simulink model "BLOC_Clutch"  (R2016a)
settings: Solver=FixedStepDiscrete  StartTime=0.0  StopTime=10.0  FixedStep=hev_dt  RelTol=1e-3
undefined symbols (not defined in the file): DiscIntNeverNeededParam, fa_clu_pos, fa_clu_pv, fa_ice_inertia, fa_max_tq_clu, hev_dt
libraries: simulink x1
settings Model: Creator=Florent  LastModifiedBy=Florent
settings OptimizationCC: DefaultParameterBehavior=Inlined  OptimizeModelRefInitCode=on  LifeSpan=1
settings RTWCC: SystemTargetFile=ert.tlc  TemplateMakefile=ert_default_tmf  GenerateReport=on  IncludeHyperlinkInReport=on  LaunchReport=on  TargetLang=C++  GenerateTraceInfo=on  GenerateTraceReport=on  GenerateTraceReportSl=on  GenerateTraceReportSf=on  GenerateTraceReportEml=on
settings CodeAppCC: ForceParamTrailComments=on  OperatorAnnotations=on  SimulinkDataObjDesc=on  SFDataObjDesc=on  MATLABFcnDesc=on  InsertBlockDesc=on  MATLABSourceComments=on
settings ERTTargetCC: GenerateSampleERTMain=on  MultiInstanceERTCode=on  CodeInterfacePackaging=C++ class  InlinedParameterPlacement=NonHierarchical  RootIOFormat=Structure reference  ERTCustomFileTemplate=example_file_process.tlc

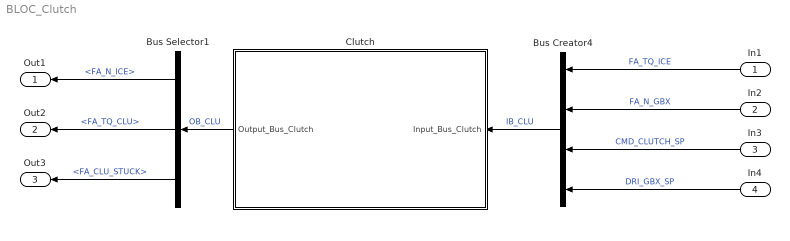
== system BLOC_Clutch ==
  In1 : Inport
  In2 : Inport  Port=2
  In3 : Inport  Port=3
  In4 : Inport  Port=4
  Bus Creator4 : BusCreator  Inputs=4
  Bus Selector1 : BusSelector  OutputSignals=FA_N_ICE,FA_TQ_CLU,FA_CLU_STUCK
  Clutch : Subsystem  TreatAsAtomicUnit=on  SystemSampleTime=hev_dt
  Out1 : Outport
  Out2 : Outport  Port=2
  Out3 : Outport  Port=3
  wires:
  In2/1 -> Bus Creator4/2  "FA_N_GBX"
  In1/1 -> Bus Creator4/1  "FA_TQ_ICE"
  In3/1 -> Bus Creator4/3  "CMD_CLUTCH_SP"
  In4/1 -> Bus Creator4/4  "DRI_GBX_SP"
  Bus Creator4/1 -> Clutch/1("Input_Bus_Clutch ")  "IB_CLU"
  Bus Selector1/2 -> Out2/1  "<FA_TQ_CLU>"
  Clutch/1(Output_Bus_Clutch) -> Bus Selector1/1  "OB_CLU"
  Bus Selector1/3 -> Out3/1  "<FA_CLU_STUCK>"
  Bus Selector1/1 -> Out1/1  "<FA_N_ICE>"

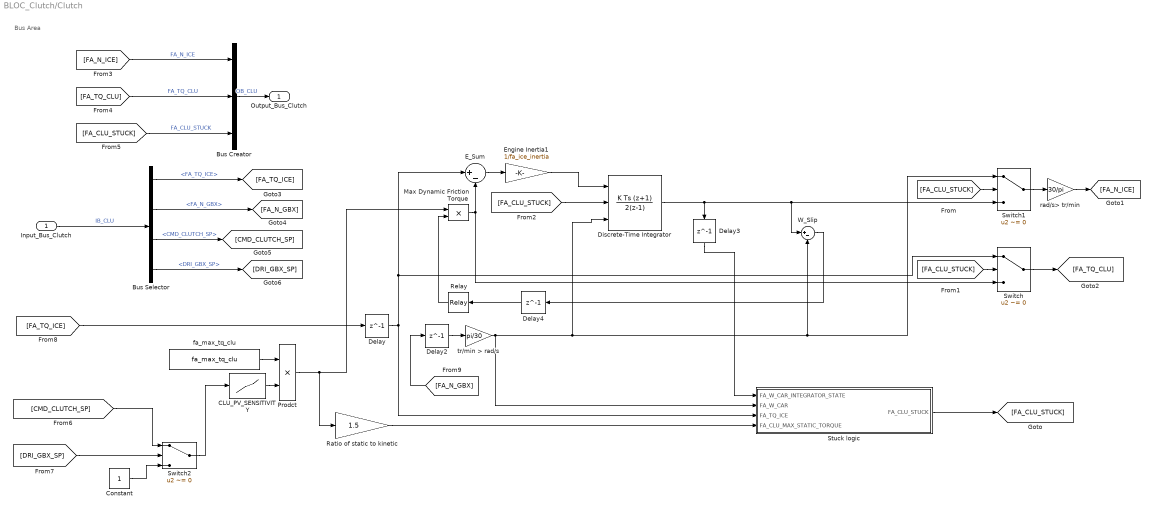
== system BLOC_Clutch/Clutch ==
  note: Bus Area
  "Input_Bus_Clutch " : Inport
  " tr/min > rad/s" : Gain  Gain=pi/30  SampleTime=hev_dt
  Bus Creator : BusCreator  Inputs=3
  Bus Selector : BusSelector  OutputSignals=FA_TQ_ICE,FA_N_GBX,CMD_CLUTCH_SP,DRI_GBX_SP
  CLU_PV_SENSITIVITY : Lookup_n-D  NumberOfTableDimensions=1  BreakpointsForDimension1=fa_clu_pv  Table=fa_clu_pos  ExtrapMethod=Clip  UseLastTableValue=on  SampleTime=hev_dt  RndMeth=Simplest  InputSameDT=on
  Constant : Constant
  Delay{,2..4} (4 alike) : Delay  DelayLength=1  SampleTime=hev_dt
  Discrete-Time Integrator : DiscreteIntegrator  IntegratorMethod=Integration: Trapezoidal  ExternalReset=falling  InitialConditionSource=external  SampleTime=hev_dt  ICPrevOutput=DiscIntNeverNeededParam  ICPrevScaledInput=DiscIntNeverNeededParam
  E_Sum : Sum  Inputs=|+-  SampleTime=hev_dt  SaturateOnIntegerOverflow=on  InputSameDT=on  OutDataTypeStr=Inherit: Same as first input
  Engine Inertia1 : Gain  Gain=1/fa_ice_inertia  SampleTime=hev_dt  SaturateOnIntegerOverflow=on  OutDataTypeStr=Inherit: Same as input  ParamDataTypeStr=Inherit: Same as input
  Max Dynamic Friction Torque : Product  SampleTime=hev_dt  SaturateOnIntegerOverflow=on  RndMeth=Zero  InputSameDT=on  OutDataTypeStr=Inherit: Same as first input
  Prodct : Product  SampleTime=hev_dt  RndMeth=Zero
  Ratio of static to kinetic : Gain  Gain=1.5  SampleTime=hev_dt  SaturateOnIntegerOverflow=on  OutDataTypeStr=Inherit: Same as input  ParamDataTypeStr=Inherit: Same as input
  Relay : Relay  OnSwitchValue=0  OffSwitchValue=0  OffOutputValue=-1  SampleTime=hev_dt
  Stuck logic : Subsystem
  Switch : Switch  Criteria=u2 ~= 0  SampleTime=hev_dt
  Switch1 : Switch  Criteria=u2 ~= 0  SampleTime=hev_dt
  Switch2 : Switch  Criteria=u2 ~= 0
  W_Slip : Sum  Inputs=|+-  SampleTime=hev_dt  SaturateOnIntegerOverflow=on  InputSameDT=on  OutDataTypeStr=Inherit: Same as first input
  fa_max_tq_clu : Constant  Value=fa_max_tq_clu
  rad/s> tr/min : Gain  Gain=30/pi  SampleTime=hev_dt
  Output_Bus_Clutch : Outport
  wires:
  [FA_TQ_ICE] -> Delay/1
  Switch1/1 -> rad/s> tr/min/1
  Switch/1 -> [FA_TQ_CLU]
  fa_max_tq_clu/1 -> Prodct/1
  Delay/1 -> E_Sum/1, Switch/1, Stuck logic/3(FA_TQ_ICE)
  " tr/min > rad/s"/1 -> Discrete-Time Integrator/3, Switch1/1, W_Slip/2, Stuck logic/2(FA_W_CAR)
  rad/s> tr/min/1 -> [FA_N_ICE]
  Ratio of static to kinetic/1 -> Stuck logic/4(FA_CLU_MAX_STATIC_TORQUE)
  E_Sum/1 -> Engine Inertia1/1
  Engine Inertia1/1 -> Discrete-Time Integrator/1
  Relay/1 -> Max Dynamic Friction Torque/2
  Max Dynamic Friction Torque/1 -> E_Sum/2, Switch/3
  [FA_CLU_STUCK] -> Switch1/2
  [FA_CLU_STUCK] -> Switch/2
  [FA_CLU_STUCK] -> Discrete-Time Integrator/2
  W_Slip/1 -> Delay4/1
  Delay2/1 -> " tr/min > rad/s"/1
  [FA_N_GBX] -> Delay2/1
  [CMD_CLUTCH_SP] -> Switch2/1
  Discrete-Time Integrator/1 -> W_Slip/1, Switch1/3, Delay3/1
  Delay3/1 -> Stuck logic/1(FA_W_CAR_INTEGRATOR_STATE)
  Switch2/1 -> CLU_PV_SENSITIVITY/1
  [DRI_GBX_SP] -> Switch2/2
  Constant/1 -> Switch2/3
  Delay4/1 -> Relay/1
  CLU_PV_SENSITIVITY/1 -> Prodct/2
  Stuck logic/1(FA_CLU_STUCK) -> [FA_CLU_STUCK]
  Bus Creator/1 -> Output_Bus_Clutch/1  "OB_CLU"
  [FA_N_ICE] -> Bus Creator/1  "FA_N_ICE"
  [FA_TQ_CLU] -> Bus Creator/2  "FA_TQ_CLU"
  [FA_CLU_STUCK] -> Bus Creator/3  "FA_CLU_STUCK"
  "Input_Bus_Clutch "/1 -> Bus Selector/1  "IB_CLU"
  Bus Selector/1 -> [FA_TQ_ICE]  "<FA_TQ_ICE>"
  Bus Selector/2 -> [FA_N_GBX]  "<FA_N_GBX>"
  Bus Selector/3 -> [CMD_CLUTCH_SP]  "<CMD_CLUTCH_SP>"
  Bus Selector/4 -> [DRI_GBX_SP]  "<DRI_GBX_SP>"
  Prodct/1 -> Ratio of static to kinetic/1, Max Dynamic Friction Torque/1

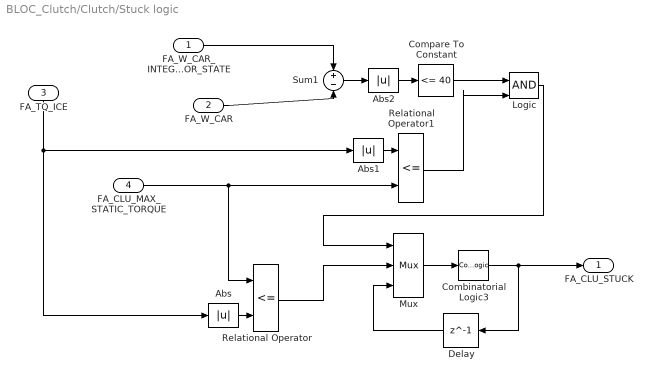
== system BLOC_Clutch/Clutch/Stuck logic ==
  FA_W_CAR_INTEGRATOR_STATE : Inport
  FA_W_CAR : Inport  Port=2
  FA_TQ_ICE : Inport  Port=3
  FA_CLU_MAX_STATIC_TORQUE : Inport  Port=4
  Abs : Abs  SampleTime=hev_dt  SaturateOnIntegerOverflow=on
  Abs1 : Abs  SampleTime=hev_dt  SaturateOnIntegerOverflow=on
  Abs2 : Abs  SampleTime=hev_dt  SaturateOnIntegerOverflow=on
  Combinatorial Logic3 : CombinatorialLogic  Description=TRUTH_TABLE_FROM_FABIEN  TruthTable=[0;1;0;0;1;1;0;1]  SampleTime=hev_dt
  Compare To Constant : simulink/Logic and Bit Operations/Compare To Constant  relop=<=  const=40  OutDataTypeStr=boolean
  Delay : Delay  DelayLength=1  SampleTime=hev_dt
  Logic : Logic  IconShape=distinctive  SampleTime=hev_dt
  Mux : Mux  Inputs=3
  Relational Operator : RelationalOperator  Operator=<=  SampleTime=hev_dt  InputSameDT=on
  Relational Operator1 : RelationalOperator  Operator=<=  SampleTime=hev_dt  InputSameDT=on
  Sum1 : Sum  Inputs=+-  SampleTime=hev_dt  SaturateOnIntegerOverflow=on  InputSameDT=on  OutDataTypeStr=Inherit: Same as first input
  FA_CLU_STUCK : Outport
  wires:
  FA_CLU_MAX_STATIC_TORQUE/1 -> Relational Operator1/2, Relational Operator/1
  Sum1/1 -> Abs2/1
  Abs1/1 -> Relational Operator1/1
  Delay/1 -> Mux/3
  Combinatorial Logic3/1 -> Delay/1, FA_CLU_STUCK/1
  Mux/1 -> Combinatorial Logic3/1
  Abs/1 -> Relational Operator/2
  Relational Operator/1 -> Mux/2
  Logic/1 -> Mux/1
  Abs2/1 -> Compare To Constant/1
  Compare To Constant/1 -> Logic/1
  Relational Operator1/1 -> Logic/2
  FA_TQ_ICE/1 -> Abs1/1, Abs/1
  FA_W_CAR_INTEGRATOR_STATE/1 -> Sum1/1
  FA_W_CAR/1 -> Sum1/2
